simulink model "slexForEachOverlapExample"  (R2017b)
settings: Solver=FixedStepAuto  StartTime=0.0  StopTime=0  RelTol=1e-3
undefined symbols (not defined in the file or in its folder): matlabroot
CloseFcn:
  | h_original = findobj('Type', 'figure', 'Name', 'For Each Demo: Original Image');
  | close(h_original);
  | h_processed = findobj('Type', 'figure', 'Name', 'For Each Demo: Processed Image');
  | close(h_processed);
  | clear h_original h_processed;
settings Model: Creator=The MathWorks, Inc.  LastModifiedBy=prave
settings DataIOCC: SaveOutput=off  DSMLogging=off  SaveTime=off
settings OptimizationCC: DefaultParameterBehavior=Inlined  EnhancedBackFolding=on  PassReuseOutputArgsAs=Individual arguments
settings DebuggingCC: ParameterTunabilityLossMsg=error
settings SFSimCC: MATLABDynamicMemAlloc=off
settings RTWCC: SystemTargetFile=ert.tlc  TemplateMakefile=ert_default_tmf  GenerateReport=on  IncludeHyperlinkInReport=on  LaunchReport=on  GenerateTraceInfo=on  GenerateTraceReport=on  GenerateTraceReportSl=on  GenerateTraceReportSf=on  GenerateTraceReportEml=on
settings CodeAppCC: ForceParamTrailComments=on  IgnoreCustomStorageClasses=off  OperatorAnnotations=on  SimulinkDataObjDesc=on  SFDataObjDesc=on  InsertBlockDesc=on
settings ERTTargetCC: TargetLangStandard=C99 (ISO)  GenerateSampleERTMain=on  InlinedParameterPlacement=NonHierarchical  ERTCustomFileTemplate=example_file_process.tlc

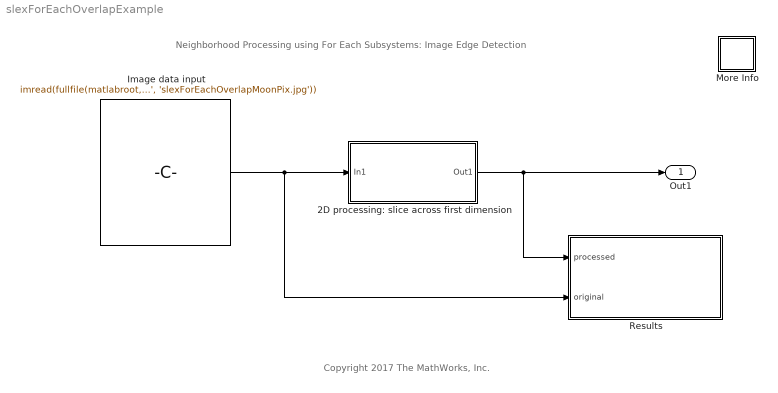
== system slexForEachOverlapExample ==
  note: Neighborhood Processing using For Each Subsystems:
      | Image Edge Detection
  note: Copyright 2017 The MathWorks, Inc.
  2D processing: slice across first dimension : Subsystem  TreatAsAtomicUnit=on
  Image data input : Constant  Value=imread(fullfile(matlabroot, 'toolbox', 'simulink', 'simdemos', 'simfeatures', 'images', 'slexForEachOverlapMoonPix.jpg'))  VectorParams1D=off
      mask Display: image(fullfile(matlabroot, 'toolbox', 'simulink', 'simdemos', 'simfeatures', 'images', 'slexForEachOverlapMoonPix.jpg'));
  More Info : Subsystem
      settings: OpenFcn=showdemo(bdroot(gcb))
      mask Display: disp('?')
  Results : MATLAB Function  TreatAsAtomicUnit=on
  Out1 : Outport
  wires:
  Image data input/1 -> Results/2(original), 2D processing: slice across first dimension/1(In1)
  2D processing: slice across first dimension/1(Out1) -> Results/1(processed), Out1/1

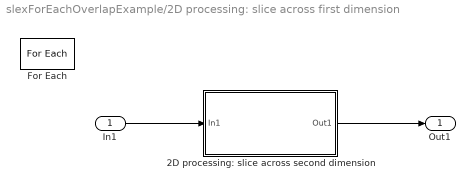
== system slexForEachOverlapExample/2D processing: slice across first dimension ==
  In1 : Inport  Partition=on  PartitionDimension=1  PartitionWidth=3  PartitionOffset=-2
  2D processing: slice across second dimension : Subsystem  TreatAsAtomicUnit=on
  For Each : ForEach  DisableCoverage=on  IndexMode=One-based
  Out1 : Outport  ConcatenationDimension=1
  wires:
  In1/1 -> 2D processing: slice across second dimension/1(In1)
  2D processing: slice across second dimension/1(Out1) -> Out1/1

== system slexForEachOverlapExample/More Info ==

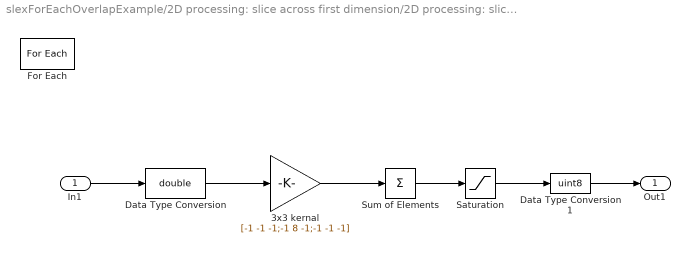
== system slexForEachOverlapExample/2D processing: slice across first dimension/2D processing: slice across second dimension ==
  In1 : Inport  Partition=on  PartitionDimension=2  PartitionWidth=3  PartitionOffset=-2
  3x3 kernal : Gain  Gain=[-1 -1 -1;-1 8 -1;-1 -1 -1]
  Data Type Conversion : DataTypeConversion  OutDataTypeStr=double
  Data Type Conversion1 : DataTypeConversion  OutDataTypeStr=uint8
  For Each : ForEach  DisableCoverage=on  IndexMode=One-based
  Saturation : Saturate  UpperLimit=255  LowerLimit=0
  Sum of Elements : Sum  Inputs=+
  Out1 : Outport  ConcatenationDimension=2
  wires:
  3x3 kernal/1 -> Sum of Elements/1
  In1/1 -> Data Type Conversion/1
  Data Type Conversion/1 -> 3x3 kernal/1
  Data Type Conversion1/1 -> Out1/1
  Sum of Elements/1 -> Saturation/1
  Saturation/1 -> Data Type Conversion1/1

== matlab function slexForEachOverlapExample/Results ==
  data: processed input; original input
function show_images(processed, original)
% Copyright 2017 The MathWorks, Inc.

coder.extrinsic('imshow');
figure('Name', 'For Each Demo: Original Image', 'NumberTitle', 'off');
imshow(original)

figure('Name', 'For Each Demo: Processed Image', 'NumberTitle', 'off');
imshow(processed);
